simulink model "B5_simulation_paparazzi"  (R2021b)
settings: Solver=VariableStepAuto  StartTime=0.0  StopTime=5.5  FixedStep=0.002  RelTol=1e-3
values from neighbouring files (symbols this model uses):
  coef_sim_1 = tf_des_d.Denominator{1}(2)    [A11_setup_script_pprz.m]    (also in A1_setup_script.m; A6_slow_actuator.m)
  coef_sim_2 = tf_des_d.Numerator{1}(2)    [A11_setup_script_pprz.m]    (also in A1_setup_script.m; A6_slow_actuator.m)
  coeff = 1    [A11_setup_script_pprz.m]    (also in A12_sim_multi_run.m = coeff_list(i))
  doublet_mag = - 0.15    (= -0.15)    [A11_setup_script_pprz.m]    (also in A1_setup_script.m)
  doublet_time = 6    [A11_setup_script_pprz.m]    (also in A1_setup_script.m)
  f_8 = 1    [A11_setup_script_pprz.m]    (also in A1_setup_script.m)
  FILT_CUTOFF = 2*pi*5    (= 31.4159265359)    [A11_setup_script_pprz.m]    (also in A1_setup_script.m)
  FILTER = 1    [A11_setup_script_pprz.m]    (also in A1_setup_script.m)
  G1 = inv(I)*G1_r    [A10_simple_plant.m]    (also in A11_setup_script_pprz.m = G1/scale; A1_setup_script.m = [G1;G1_T])
  G2 = G2/scale    [A11_setup_script_pprz.m]    (also in A1_setup_script.m = (1/sampling_time)*inv(I)*(G2_r))
  h_plate = 0.3    [A11_setup_script_pprz.m]    (also in A1_setup_script.m = 0.16)
  I = eye(3,3)    [A10_simple_plant.m]    (also in A11_setup_script_pprz.m; A1_setup_script.m; A2_B_matrix_generation_symbolic.m = [Ixx 0 0; A3_B_matrix_generation_symbolic_cascaded.m = [Ixx 0 0)
  Iyy = 0.0008    [A11_setup_script_pprz.m]    (also in A1_setup_script.m = 0.0015)
  K = 7    [A11_setup_script_pprz.m]    (also in A1_setup_script.m = 10)
  K_act = 50    [A10_simple_plant.m]    (also in A11_setup_script_pprz.m = 20; A1_setup_script.m = 20)
  K_d = 15    [A11_setup_script_pprz.m]    (also in A1_setup_script.m = 25)
  K_dd = K_act    (= 20)    [A11_setup_script_pprz.m]    (also in A1_setup_script.m)
  K_ec = 50    [A11_setup_script_pprz.m]    (also in A1_setup_script.m = 251)
  K_ec_d = 13    [A11_setup_script_pprz.m]    (also in A1_setup_script.m = 25)
  K_ec_d_u = 1.5    [A11_setup_script_pprz.m]    (also in A1_setup_script.m = 5)
  K_ec_d_v = 1.5    [A11_setup_script_pprz.m]    (also in A1_setup_script.m = 5)
  K_ec_dd = 9    [A11_setup_script_pprz.m]    (also in A1_setup_script.m = 45)
  K_ec_i = 0    [A11_setup_script_pprz.m]    (also in A1_setup_script.m = 380)
  K_ec_u = 1.5    [A11_setup_script_pprz.m]    (also in A1_setup_script.m = 5)
  K_ec_v = 1.5    [A11_setup_script_pprz.m]    (also in A1_setup_script.m = 5)
  K_t = 0.0005    [A10_simple_plant.m]    (also in A11_setup_script_pprz.m = 6.557e-08; A1_setup_script.m = 6.557e-08)
  K_u = 1.0    (= 1)    [A11_setup_script_pprz.m]    (also in A1_setup_script.m = 1.5)
  K_u_d = 2.5    [A11_setup_script_pprz.m]    (also in A1_setup_script.m = 7)
  K_v = 1.0    (= 1)    [A11_setup_script_pprz.m]    (also in A1_setup_script.m = 1.5)
  K_v_d = 2.5    [A11_setup_script_pprz.m]    (also in A1_setup_script.m = 7)
  K_w = 1.0    (= 1)    [A11_setup_script_pprz.m]    (also in A1_setup_script.m = 4.5)
  K_w_d = 2.5    [A11_setup_script_pprz.m]    (also in A1_setup_script.m = 7)
  l_plate = 0.1    [A11_setup_script_pprz.m]    (also in A1_setup_script.m = 0.11)
  m = 0.4    [A10_simple_plant.m]    (also in A11_setup_script_pprz.m; A1_setup_script.m)
  NOISE = 0    [A11_setup_script_pprz.m]    (also in A1_setup_script.m)
  NOISE_ACC = 0.00005    (= 5e-05)    [A11_setup_script_pprz.m]    (also in A1_setup_script.m)
  NOISE_GYRO = 0.00005    (= 5e-05)    [A11_setup_script_pprz.m]    (also in A1_setup_script.m)
  NOISE_RPM = 200    [A11_setup_script_pprz.m]    (also in A1_setup_script.m)
  omega_des = 20.00    (= 20)    [A11_setup_script_pprz.m]    (also in A1_setup_script.m; A6_slow_actuator.m = 49)
  sampling_time = 1/frequency    (= 0.002)    [A11_setup_script_pprz.m]    (also in A12_sim_multi_run.m; A1_setup_script.m; A6_slow_actuator.m)
  scale_8 = 1.6    [A11_setup_script_pprz.m]    (also in A1_setup_script.m)
  start_8 = 2    [A11_setup_script_pprz.m]    (also in A1_setup_script.m)
  start_time = 2    [A11_setup_script_pprz.m]    (also in A1_setup_script.m = 1)
  t_8 = 10    [A11_setup_script_pprz.m]    (also in A1_setup_script.m)
  w_plate = 0.3    [A11_setup_script_pprz.m]    (also in A1_setup_script.m = 0.36)
undefined symbols (not defined in the file or in its folder): DiscIntNeverNeededParam
libraries: simulink x11, cstblocks x9, dspinverses x8, dspmathops x4, dspstat3 x4, aerolibutil x3, sharedutil x2, aerolibanim x1
(part 2 of 5)

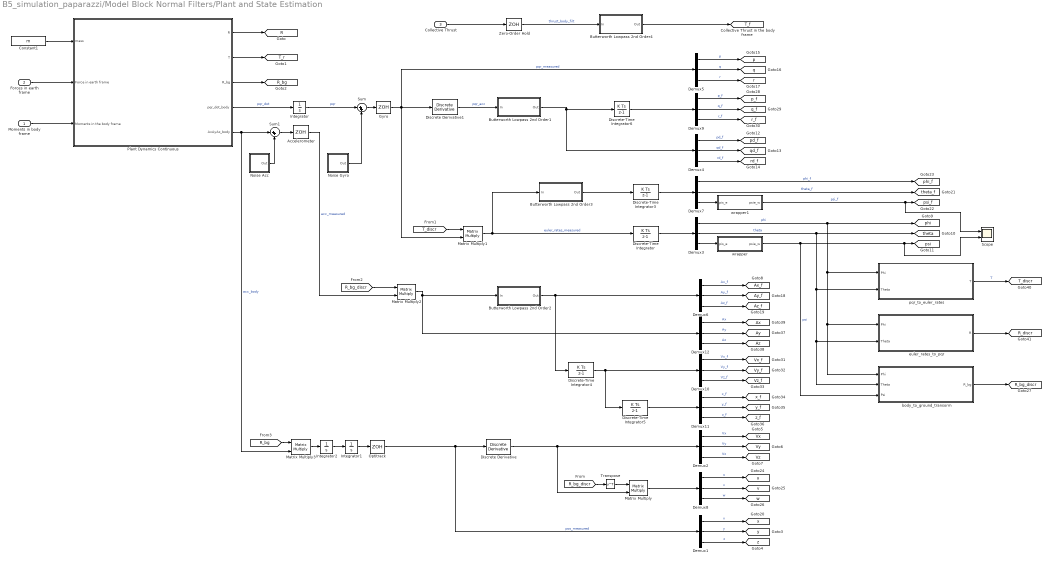
== system B5_simulation_paparazzi/Model Block Normal Filters/Plant and State Estimation ==
  Moments in body frame : Inport
  Forces in earth frame : Inport  Port=2
  Collective Thrust : Inport  Port=3
  Accelerometer : ZeroOrderHold  SampleTime=sampling_time
  Butterworth Lowpass 2nd Order1 : Subsystem
  Butterworth Lowpass 2nd Order2 : Subsystem
  Butterworth Lowpass 2nd Order3 : Subsystem
  Butterworth Lowpass 2nd Order4 : Subsystem
  Constant1 : Constant  Value=m  SampleTime=sampling_time
  Demux{1..12} (12 alike) : Demux  Outputs=3
  Discrete Derivative : simulink/Discrete/Discrete Derivative  gainval=1.0  ICPrevScaledInput=0.0  OutMin=[]  OutMax=[]  OutDataType=fixdt(1, 16)  OutScaling=2^-10  DoSatur=off
  Discrete Derivative1 : simulink/Discrete/Discrete Derivative  gainval=1.0  ICPrevScaledInput=0.0  OutMin=[]  OutMax=[]  OutDataType=fixdt(1, 16)  OutScaling=2^-10  DoSatur=off
  Discrete-Time Integrator{,3..5} (4 alike) : DiscreteIntegrator  SampleTime=sampling_time  ICPrevOutput=DiscIntNeverNeededParam  ICPrevScaledInput=DiscIntNeverNeededParam
  Discrete-Time Integrator6 : DiscreteIntegrator  SampleTime=-1  ICPrevOutput=DiscIntNeverNeededParam  ICPrevScaledInput=DiscIntNeverNeededParam
  Gyro : ZeroOrderHold  SampleTime=sampling_time
  Integrator : Integrator
  Integrator1 : Integrator
  Integrator2 : Integrator
  Matrix Multiply{,1..3} (4 alike) : Product  Multiplication=Matrix(*)
  Noise Acc : Subsystem
  Noise Gyro : Subsystem
  Optitrack : ZeroOrderHold  SampleTime=sampling_time
  Plant Dynamics Continuous : Subsystem
  Scope : Scope  NumInputPorts=2
  Sum : Sum  Inputs=|++
  Sum1 : Sum  Inputs=|++
  Transpose : Math  Operator=transpose  SaturateOnIntegerOverflow=on
  Zero-Order Hold : ZeroOrderHold  SampleTime=sampling_time
  body_to_ground_transorm : MATLAB Function  Description=|  TreatAsAtomicUnit=on
      | This function computes the rotational matrix to pass from the body frame to the world frame. 
      | Takes as inpout the euler angles.
  euler_rates_to_pqr : MATLAB Function  TreatAsAtomicUnit=on
  pqr_to_euler_rates : MATLAB Function  TreatAsAtomicUnit=on
  wrapper : MATLAB Function  TreatAsAtomicUnit=on
  wrapper1 : MATLAB Function  TreatAsAtomicUnit=on
  tag scope: Ax=global, Ax_f=global, Ay=global, Ay_f=global, Az=global, Az_f=global, R=global, R_bg=global, R_bg_discr=global, R_discr=global, T_discr=global, T_f=global, T_r=global, Vx=global, Vx_f=global, Vy=global, Vy_f=global, Vz=global, Vz_f=global, p=global, p_f=global, pd_f=global, phi=global, phi_f=global, psi=global, psi_f=global, q=global, q_f=global, qd_f=global, r=global, r_f=global, rd_f=global, theta=global, theta_f=global, u=global, v=global, w=global, x=global, x_f=global, y=global, y_f=global, z=global, z_f=global
  wires:
  Demux3/2 -> euler_rates_to_pqr/2(Theta), body_to_ground_transorm/2(Theta), pqr_to_euler_rates/2(Theta), [theta]  "theta"
  Demux4/1 -> [pd_f]  "pd_f"
  Demux3/1 -> body_to_ground_transorm/1(Phi), euler_rates_to_pqr/1(Phi), pqr_to_euler_rates/1(Phi), [phi]  "phi"
  Demux4/2 -> [qd_f]  "qd_f"
  Demux3/3 -> wrapper/1(pis_e)
  Discrete-Time Integrator/1 -> Demux3/1
  Demux5/2 -> [q]  "q"
  Demux5/1 -> [p]  "p"
  Plant Dynamics Continuous/4(pqr_dot_body) -> Integrator/1  "pqr_dot"
  Demux5/3 -> [r]  "r"
  Integrator/1 -> Sum/1  "pqr"
  Butterworth Lowpass 2nd Order1/1(Out) -> Demux4/1, Discrete-Time Integrator6/1
  Demux4/3 -> [rd_f]  "rd_f"
  Moments in body frame/1 -> Plant Dynamics Continuous/3(Moments in the body frame)
  Constant1/1 -> Plant Dynamics Continuous/1(mass)
  Forces in earth frame/1 -> Plant Dynamics Continuous/2(Force in earth frame)
  Plant Dynamics Continuous/1(R) -> [R]
  Plant Dynamics Continuous/2(T) -> [T_r]
  Plant Dynamics Continuous/3(R_bg) -> [R_bg]
  Demux2/2 -> [Vy]  "Vy"
  Demux6/2 -> [Ay_f]  "Ay_f"
  Discrete Derivative/1 -> Demux2/1, Matrix Multiply/2
  Demux6/1 -> [Ax_f]  "Ax_f"
  Accelerometer/1 -> Matrix Multiply2/2  "acc_measured"
  Demux2/1 -> [Vx]  "Vx"
  Demux1/2 -> [y]  "y"
  Demux1/1 -> [x]  "x"
  Demux1/3 -> [z]  "z"
  Demux6/3 -> [Az_f]  "Az_f"
  Demux2/3 -> [Vz]  "Vz"
  Plant Dynamics Continuous/5(AxAyAz_body) -> Matrix Multiply3/2, Sum1/1  "acc_body"
  Demux7/3 -> wrapper1/1(pis_e)
  Demux7/1 -> [phi_f]  "phi_f"
  Demux7/2 -> [theta_f]  "theta_f"
  Discrete-Time Integrator3/1 -> Demux7/1
  [R_bg_discr] -> Transpose/1
  Transpose/1 -> Matrix Multiply/1
  Demux8/2 -> [v]  "v"
  Demux8/1 -> [u]  "u"
  Demux8/3 -> [w]  "w"
  Matrix Multiply/1 -> Demux8/1
  Zero-Order Hold/1 -> Butterworth Lowpass 2nd Order4/1(In)  "thrust_body_filt"
  Collective Thrust/1 -> Zero-Order Hold/1
  Demux9/3 -> [r_f]  "r_f"
  Demux9/1 -> [p_f]  "p_f"
  Demux9/2 -> [q_f]  "q_f"
  Demux10/1 -> [Vx_f]  "Vx_f"
  Demux10/2 -> [Vy_f]  "Vy_f"
  Demux10/3 -> [Vz_f]  "Vz_f"
  Demux11/2 -> [y_f]  "y_f"
  Discrete-Time Integrator5/1 -> Demux11/1
  Demux11/1 -> [x_f]  "x_f"
  Demux11/3 -> [z_f]  "z_f"
  Discrete-Time Integrator4/1 -> Demux10/1, Discrete-Time Integrator5/1
  Demux12/2 -> [Ay]  "Ay"
  Demux12/1 -> [Ax]  "Ax"
  Demux12/3 -> [Az]  "Az"
  [T_discr] -> Matrix Multiply1/1
  Matrix Multiply1/1 -> Butterworth Lowpass 2nd Order3/1(In), Discrete-Time Integrator/1  "euler_rates_measured"
  euler_rates_to_pqr/1(R) -> [R_discr]
  pqr_to_euler_rates/1(T) -> [T_discr]  "T"
  body_to_ground_transorm/1(R_bg) -> [R_bg_discr]
  wrapper/1(psie_w) -> body_to_ground_transorm/3(Psi), Scope/2, [psi]  "psi"
  wrapper1/1(psie_w) -> Scope/1, [psi_f]  "psi_f"
  Sum/1 -> Gyro/1
  Sum1/1 -> Accelerometer/1
  Butterworth Lowpass 2nd Order2/1(Out) -> Discrete-Time Integrator4/1, Demux6/1
  [R_bg_discr] -> Matrix Multiply2/1
  Matrix Multiply2/1 -> Butterworth Lowpass 2nd Order2/1(In), Demux12/1
  Discrete Derivative1/1 -> Butterworth Lowpass 2nd Order1/1(In)  "pqr_acc"
  Discrete-Time Integrator6/1 -> Demux9/1
  Gyro/1 -> Demux5/1, Discrete Derivative1/1, Matrix Multiply1/2  "pqr_measured"
  Integrator1/1 -> Optitrack/1
  Integrator2/1 -> Integrator1/1
  Optitrack/1 -> Demux1/1, Discrete Derivative/1  "pos_measured"
  Matrix Multiply3/1 -> Integrator2/1
  [R_bg] -> Matrix Multiply3/1
  Noise Acc/1(Out) -> Sum1/2
  Noise Gyro/1(Out) -> Sum/2
  Butterworth Lowpass 2nd Order3/1(Out) -> Discrete-Time Integrator3/1
  Butterworth Lowpass 2nd Order4/1(Out) -> [T_f]

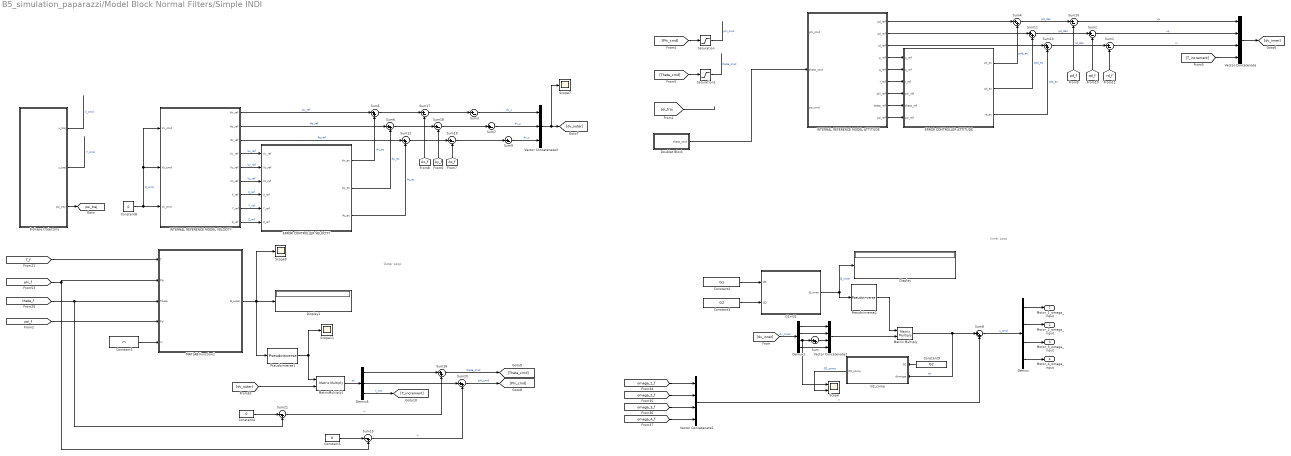
== system B5_simulation_paparazzi/Model Block Normal Filters/Simple INDI ==
  note: Inner Loop
  note: Outer Loop
  8-shape trajectory : Subsystem
  Constant1 : Constant  Value=m  SampleTime=sampling_time
  Constant2 : Constant  Value=G1  SampleTime=sampling_time
  Constant3 : Constant  Value=G2  SampleTime=sampling_time
  Constant4 : Constant  Value=0
  Constant5 : Constant  Value=0
  Constant8 : Constant  Value=0  SampleTime=sampling_time
  Constant9 : Constant  Value=G2  SampleTime=sampling_time
  Demux : Demux
  Demux1 : Demux
  Demux5 : Demux  Outputs=3
  Display : Display
  Display1 : Display
  Doublet Block : Subsystem
  ERROR CONTROLLER ATTITUDE : Subsystem
  ERROR CONTROLLER VELOCITY : Subsystem
  G1+G2 : MATLAB Function  TreatAsAtomicUnit=on
  G2_comp : MATLAB Function  TreatAsAtomicUnit=on
  INTERNAL REFERENCE MODEL ATTITUDE : Subsystem
  INTERNAL REFERENCE MODEL VELOCITY : Subsystem
  MATLAB Function1 : MATLAB Function  TreatAsAtomicUnit=on
  Matrix Multiply : Product  Multiplication=Matrix(*)
  MatrixMultiply1 : Product  Multiplication=Matrix(*)
  Pseudoinverse1 : dspinverses/Pseudoinverse  wanterr=off  SimulateUsing=Interpreted execution
      settings: SourceProductBaseCode=DS
  Pseudoinverse2 : dspinverses/Pseudoinverse  wanterr=off  SimulateUsing=Interpreted execution
      settings: SourceProductBaseCode=DS
  Saturation : Saturate
  Saturation1 : Saturate
  Scope : Scope  NumInputPorts=2
  Scope11 : Scope
  Scope7 : Scope
  Scope9 : Scope
  Sum{,4..6,8,11..13,16,20} (10 alike) : Sum  Inputs=|++
  Sum{1..3,7,9..10,17..19} (9 alike) : Sum  Inputs=|+-
  Sum15 : Sum  Inputs=|-+
  Sum21 : Sum  Inputs=|-+
  Vector Concatenate : Concatenate  NumInputs=4
  Vector Concatenate1 : Concatenate  NumInputs=4
  Vector Concatenate2 : Concatenate  NumInputs=4
  Vector Concatenate3 : Concatenate  NumInputs=3
  Motor_1_omega_input : Outport
  Motor_2_omega_input : Outport  Port=2
  Motor_3_omega_input : Outport  Port=3
  Motor_4_omega_input : Outport  Port=4
  tag scope: psi_traj=global
  wires:
  G1+G2/1(B_inner) -> Pseudoinverse2/1, Display/1  "B_inner"
  Vector Concatenate1/1 -> Sum8/2  "u"
  Vector Concatenate/1 -> [dv_inner]
  Matrix Multiply/1 -> G2_comp/2(domega), Sum8/1  "du"
  Demux/1 -> Motor_1_omega_input/1
  [omega_4_f] -> Vector Concatenate1/4
  [omega_2_f] -> Vector Concatenate1/2
  Demux/3 -> Motor_3_omega_input/1
  Sum8/1 -> Demux/1  "u_cmd"
  Pseudoinverse2/1 -> Matrix Multiply/1
  [omega_1_f] -> Vector Concatenate1/1
  Demux/2 -> Motor_2_omega_input/1
  Demux/4 -> Motor_4_omega_input/1
  [omega_3_f] -> Vector Concatenate1/3
  INTERNAL REFERENCE MODEL VELOCITY/5(Vy_ref) -> ERROR CONTROLLER VELOCITY/2(Vy_ref)  "Vy_ref"
  Constant4/1 -> Sum21/1
  Sum16/1 -> [Theta_cmd]  "theta_cmd"
  Sum9/1 -> Vector Concatenate3/3  "dv_z"
  INTERNAL REFERENCE MODEL VELOCITY/2(Ay_ref) -> Sum6/1  "Ay_ref"
  Sum21/1 -> Sum16/2  "u"
  INTERNAL REFERENCE MODEL VELOCITY/6(Vz_ref) -> ERROR CONTROLLER VELOCITY/3(Vz_ref)  "Vz_ref"
  INTERNAL REFERENCE MODEL VELOCITY/4(Vx_ref) -> ERROR CONTROLLER VELOCITY/1(Vx_ref)  "Vx_ref"
  ERROR CONTROLLER VELOCITY/2(Ay_ec) -> Sum6/2  "Ay_ec"
  8-shape trajectory/1(x_traj) -> ?  "X_cmd"
  Sum7/1 -> Vector Concatenate3/2  "dv_y"
  ERROR CONTROLLER VELOCITY/1(Ax_ec) -> Sum5/2  "Ax_ec"
  Sum3/1 -> Vector Concatenate3/1  "dv_x"
  ERROR CONTROLLER VELOCITY/3(Az_ec) -> Sum12/2  "Az_ec"
  Sum12/1 -> Sum19/1
  Constant8/1 -> INTERNAL REFERENCE MODEL VELOCITY/1(Vx_cmd), INTERNAL REFERENCE MODEL VELOCITY/2(Vy_cmd), INTERNAL REFERENCE MODEL VELOCITY/3(Vz_cmd)  "Z_cmd"
  Pseudoinverse1/1 -> Scope11/1, MatrixMultiply1/1
  Sum15/1 -> Sum20/2  "u"
  Vector Concatenate3/1 -> Scope7/1, [dv_outer]
  INTERNAL REFERENCE MODEL VELOCITY/1(Ax_ref) -> Sum5/1  "Ax_ref"
  INTERNAL REFERENCE MODEL VELOCITY/3(Az_ref) -> Sum12/1  "Az_ref"
  Sum20/1 -> [Phi_cmd]  "phi_cmd"
  [T_f] -> MATLAB Function1/1(T)
  Sum6/1 -> Sum18/1
  Constant5/1 -> Sum15/1
  [dv_outer] -> MatrixMultiply1/2
  MATLAB Function1/1(B_outer) -> Scope9/1, Display1/1, Pseudoinverse1/1
  Demux5/3 -> [T_increment]  "t_incr"
  MatrixMultiply1/1 -> Demux5/1  "du"
  8-shape trajectory/2(y_traj) -> ?  "Y_cmd"
  [Ax_f] -> Sum17/2
  [Ay_f] -> Sum18/2
  [Az_f] -> Sum19/2
  [Phi_cmd] -> Saturation/1
  [theta_f] -> Sum21/2, MATLAB Function1/3(Theta)
  [phi_f] -> Sum15/2, MATLAB Function1/2(Phi)
  INTERNAL REFERENCE MODEL ATTITUDE/4(p_ref) -> ERROR CONTROLLER ATTITUDE/1(p_ref)
  ERROR CONTROLLER ATTITUDE/3(rd_ec) -> Sum13/2  "rdd_ec"
  ERROR CONTROLLER ATTITUDE/2(qd_ec) -> Sum11/2  "qdd_ec"
  INTERNAL REFERENCE MODEL ATTITUDE/8(theta_ref) -> ERROR CONTROLLER ATTITUDE/5(theta_ref)
  INTERNAL REFERENCE MODEL ATTITUDE/5(q_ref) -> ERROR CONTROLLER ATTITUDE/2(q_ref)
  ERROR CONTROLLER ATTITUDE/1(pd_ec) -> Sum4/2  "pdd_ec"
  INTERNAL REFERENCE MODEL ATTITUDE/7(phi_ref) -> ERROR CONTROLLER ATTITUDE/4(phi_ref)
  INTERNAL REFERENCE MODEL ATTITUDE/9(psi_ref) -> ERROR CONTROLLER ATTITUDE/6(psi_ref)
  INTERNAL REFERENCE MODEL ATTITUDE/6(r_ref) -> ERROR CONTROLLER ATTITUDE/3(r_ref)
  [T_increment] -> Vector Concatenate/4
  Constant3/1 -> G1+G2/2(G2)
  Constant2/1 -> G1+G2/1(G1)
  Constant9/1 -> G2_comp/1(G2)
  [dv_inner] -> Demux1/1  "dv_inner"
  Sum/1 -> Vector Concatenate2/3
  Demux1/3 -> Scope/1, Sum/1
  Demux1/2 -> Vector Concatenate2/2
  Demux1/1 -> Vector Concatenate2/1
  Demux1/4 -> Vector Concatenate2/4
  Vector Concatenate2/1 -> Matrix Multiply/2
  G2_comp/1(G2_comp) -> Scope/2  "G2_comp"
  Sum5/1 -> Sum17/1
  Saturation1/1 -> ?  "theta_cmd"
  8-shape trajectory/3(psi_traj) -> [psi_traj]
  [Theta_cmd] -> Saturation1/1
  Saturation/1 -> ?  "phi_cmd"
  Sum17/1 -> Sum3/1
  Sum18/1 -> Sum7/1
  Sum19/1 -> Sum9/1
  Constant1/1 -> MATLAB Function1/5(m)
  Demux5/2 -> Sum20/1
  Demux5/1 -> Sum16/1
  [psi_f] -> MATLAB Function1/4(Psi)
  [psi_traj] -> ?
  INTERNAL REFERENCE MODEL VELOCITY/7(X_ref) -> ERROR CONTROLLER VELOCITY/4(X_ref)  "X_ref"
  INTERNAL REFERENCE MODEL VELOCITY/8(Y_ref) -> ERROR CONTROLLER VELOCITY/5(Y_ref)  "Y_ref"
  INTERNAL REFERENCE MODEL VELOCITY/9(Z_ref) -> ERROR CONTROLLER VELOCITY/6(Z_ref)  "Z_ref"
  Doublet Block/1(theta_cmd) -> INTERNAL REFERENCE MODEL ATTITUDE/2(theta_cmd)
  INTERNAL REFERENCE MODEL ATTITUDE/3(rd_ref) -> Sum13/1
  INTERNAL REFERENCE MODEL ATTITUDE/2(qd_ref) -> Sum11/1
  INTERNAL REFERENCE MODEL ATTITUDE/1(pd_ref) -> Sum4/1
  Sum11/1 -> Sum2/1  "qd_des"
  Sum4/1 -> Sum10/1  "pd_des"
  Sum10/1 -> Vector Concatenate/1  "vp"
  Sum2/1 -> Vector Concatenate/2  "vq"
  Sum1/1 -> Vector Concatenate/3  "vr"
  Sum13/1 -> Sum1/1  "rd_des"
  [pd_f] -> Sum10/2
  [qd_f] -> Sum2/2
  [rd_f] -> Sum1/2

== system B5_simulation_paparazzi/Model Block Complementary Filters/Continuous Actuator Dynamics/Noise RPM ==
  Constant : Constant  Value=NOISE  SampleTime=sampling_time
  Merge : Merge
  Switch Case : SwitchCase
  Switch Case Action Subsystem : Subsystem  TreatAsAtomicUnit=on
  Switch Case Action Subsystem1 : Subsystem  TreatAsAtomicUnit=on
  Out : Outport
  wires:
  Switch Case/2 -> Switch Case Action Subsystem1/Action
  Merge/1 -> Out/1
  Switch Case/1 -> Switch Case Action Subsystem/Action
  Constant/1 -> Switch Case/1
  Switch Case Action Subsystem1/1(Out1) -> Merge/2
  Switch Case Action Subsystem/1(Out1) -> Merge/1

== system B5_simulation_paparazzi/Model Block Complementary Filters/Extended INDI/8-shape trajectory ==
  Abs : Abs
  Abs1 : Abs
  Clock : Clock
      settings: Decimation=100
  Constant : Constant  Value=f_8
  Constant1 : Constant  Value=scale_8
  Constant2 : Constant  Value=t_8
  Constant3 : Constant  Value=sampling_time
  Constant4 : Constant  Value=0
  Constant5 : Constant  Value=start_8
  Constant6 : Constant  Value=t_8
  Constant7 : Constant  Value=start_8
  Integrator : Integrator
  MATLAB Function : MATLAB Function  TreatAsAtomicUnit=on
  Scope : Scope
  Scope1 : Scope
  Sum : Sum  Inputs=|+-
  Sum3 : Sum  Inputs=|+-
  Sum7 : Sum  Inputs=|+-
  Sum9 : Sum  Inputs=|++
  Switch : Switch  Criteria=u2 > Threshold  Threshold=t_8
  Switch1 : Switch  Criteria=u2 > Threshold  Threshold=start_8
  Zero-Order Hold : ZeroOrderHold  SampleTime=sampling_time
  x_traj : Outport
  y_traj : Outport  Port=2
  psi_traj : Outport  Port=3
  wires:
  Constant2/1 -> Switch/1
  Switch/1 -> Scope/1, MATLAB Function/1(t)  "t"
  Constant/1 -> MATLAB Function/2(f)
  MATLAB Function/2(y) -> y_traj/1, Sum7/2  "y_traj"
  Zero-Order Hold/1 -> Switch/2, Switch/3
  Constant1/1 -> MATLAB Function/3(scale)
  Constant3/1 -> MATLAB Function/4(sampling_time)
  MATLAB Function/1(x) -> x_traj/1, Sum3/2  "x_traj"
  MATLAB Function/3(psi) -> psi_traj/1  "psi_traj"
  Clock/1 -> Sum/1, Switch1/2
  Constant4/1 -> Switch1/3
  Switch1/1 -> Zero-Order Hold/1
  Constant5/1 -> Sum/2
  Sum/1 -> Switch1/1
  Constant6/1 -> MATLAB Function/5(total_time)
  Sum7/1 -> Abs1/1
  Abs/1 -> Sum9/1
  Abs1/1 -> Sum9/2
  [y] -> Sum7/1
  Sum9/1 -> Integrator/1
  Integrator/1 -> Scope1/1  "pos_err"
  [x] -> Sum3/1
  Sum3/1 -> Abs/1
  Constant7/1 -> MATLAB Function/6(start_time)

== system B5_simulation_paparazzi/Model Block Complementary Filters/Extended INDI/Doublet Block ==
  Scope : Scope
  Step : Step  Time=start_time  After=doublet_mag  SampleTime=sampling_time
  theta_cmd : Outport
  wires:
  Step/1 -> theta_cmd/1, Scope/1

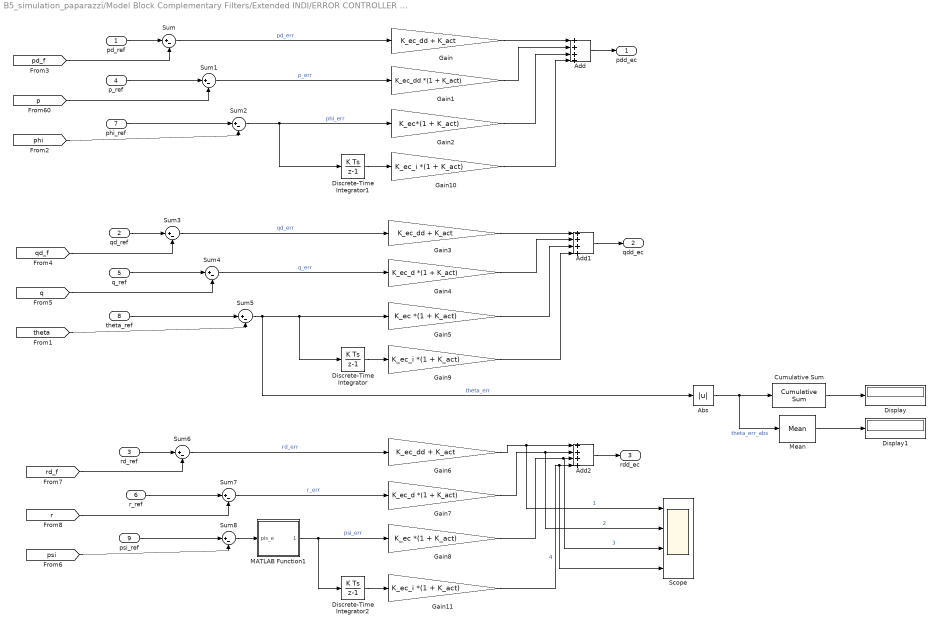
== system B5_simulation_paparazzi/Model Block Complementary Filters/Extended INDI/ERROR CONTROLLER ATTITUDE ==
  pd_ref : Inport
  qd_ref : Inport  Port=2
  rd_ref : Inport  Port=3
  p_ref : Inport  Port=4
  q_ref : Inport  Port=5
  r_ref : Inport  Port=6
  phi_ref : Inport  Port=7
  theta_ref : Inport  Port=8
  psi_ref : Inport  Port=9
  Abs : Abs
  Add : Sum  Inputs=++++
  Add1 : Sum  Inputs=++++
  Add2 : Sum  Inputs=++++
  Cumulative Sum : dspmathops/Cumulative Sum  dim=Channels (running sum)  InputProcessing=Columns as channels (frame based)  reset_popup=None  roundingMode=Floor  overflowMode=off  outputDataTypeStr=Inherit: Same as accumulator  outputMin=[]  outputMax=[]  outputLastDataTypeStr=Inherit: Same as accumulator
  Discrete-Time Integrator : DiscreteIntegrator  SampleTime=-1  ICPrevOutput=DiscIntNeverNeededParam  ICPrevScaledInput=DiscIntNeverNeededParam
  Discrete-Time Integrator1 : DiscreteIntegrator  SampleTime=-1  ICPrevOutput=DiscIntNeverNeededParam  ICPrevScaledInput=DiscIntNeverNeededParam
  Discrete-Time Integrator2 : DiscreteIntegrator  SampleTime=-1  ICPrevOutput=DiscIntNeverNeededParam  ICPrevScaledInput=DiscIntNeverNeededParam
  Display : Display
  Display1 : Display
  Gain : Gain  Gain=K_ec_dd + K_act
  Gain1 : Gain  Gain=K_ec_dd *(1 + K_act)
  Gain10 : Gain  Gain=K_ec_i *(1 + K_act)
  Gain11 : Gain  Gain=K_ec_i *(1 + K_act)
  Gain2 : Gain  Gain=K_ec*(1 + K_act)
  Gain3 : Gain  Gain=K_ec_dd + K_act
  Gain4 : Gain  Gain=K_ec_d *(1 + K_act)
  Gain5 : Gain  Gain=K_ec *(1 + K_act)
  Gain6 : Gain  Gain=K_ec_dd + K_act
  Gain7 : Gain  Gain=K_ec_d *(1 + K_act)
  Gain8 : Gain  Gain=K_ec *(1 + K_act)
  Gain9 : Gain  Gain=K_ec_i *(1 + K_act)
  MATLAB Function1 : MATLAB Function  TreatAsAtomicUnit=on
  Mean : dspstat3/Mean  run=off  InputProcessing=Columns as channels (frame based)  reset_popup=None  directionMode=Each column  dimension=1  roiEnable=off  roiType=Rectangles  roiPortion=Entire ROI  roiOutput=Individual statistics for each ROI  roiFlag=off  roundingMode=Floor  overflowMode=off  outputDataTypeStr=Inherit: Same as accumulator  outputMin=[]  outputMax=[]  outputLastDataTypeStr=Inherit: Same as accumulator
  Scope : Scope  NumInputPorts=4
  Sum{,1..8} (9 alike) : Sum  Inputs=|+-
  pdd_ec : Outport
  qdd_ec : Outport  Port=2
  rdd_ec : Outport  Port=3
  wires:
  pd_ref/1 -> Sum/1
  p_ref/1 -> Sum1/1
  Add/1 -> pdd_ec/1
  [p] -> Sum1/2
  [phi] -> Sum2/2
  phi_ref/1 -> Sum2/1
  [pd_f] -> Sum/2
  Sum/1 -> Gain/1  "pd_err"
  Gain/1 -> Add/1
  Sum1/1 -> Gain1/1  "p_err"
  Sum2/1 -> Discrete-Time Integrator1/1, Gain2/1  "phi_err"
  Gain1/1 -> Add/2
  Gain2/1 -> Add/3
  Sum4/1 -> Gain4/1  "q_err"
  [qd_f] -> Sum3/2
  Gain4/1 -> Add1/2
  Gain5/1 -> Add1/3
  theta_ref/1 -> Sum5/1
  [theta] -> Sum5/2
  [q] -> Sum4/2
  Gain3/1 -> Add1/1
  q_ref/1 -> Sum4/1
  Add1/1 -> qdd_ec/1
  qd_ref/1 -> Sum3/1
  Sum7/1 -> Gain7/1  "r_err"
  Sum8/1 -> MATLAB Function1/1(pis_e)
  Sum6/1 -> Gain6/1  "rd_err"
  [rd_f] -> Sum6/2
  Gain7/1 -> Scope/2, Add2/2  "2"
  Gain8/1 -> Scope/3, Add2/3  "3"
  psi_ref/1 -> Sum8/1
  [psi] -> Sum8/2
  [r] -> Sum7/2
  Gain6/1 -> Add2/1, Scope/1  "1"
  r_ref/1 -> Sum7/1
  Add2/1 -> rdd_ec/1
  rd_ref/1 -> Sum6/1
  Sum3/1 -> Gain3/1  "qd_err"
  Sum5/1 -> Abs/1, Discrete-Time Integrator/1, Gain5/1  "theta_err"
  MATLAB Function1/1(psie_w) -> Discrete-Time Integrator2/1, Gain8/1  "psi_err"
  Abs/1 -> Mean/1, Cumulative Sum/1  "theta_err_abs"
  Cumulative Sum/1 -> Display/1
  Mean/1 -> Display1/1
  Discrete-Time Integrator/1 -> Gain9/1
  Gain9/1 -> Add1/4
  Discrete-Time Integrator1/1 -> Gain10/1
  Gain10/1 -> Add/4
  Discrete-Time Integrator2/1 -> Gain11/1
  Gain11/1 -> Scope/4, Add2/4  "4"

== system B5_simulation_paparazzi/Model Block Complementary Filters/Extended INDI/ERROR CONTROLLER VELOCITY ==
  Vx_ref : Inport
  Vy_ref : Inport  Port=2
  Vz_ref : Inport  Port=3
  X_ref : Inport  Port=4
  Y_ref : Inport  Port=5
  Z_ref : Inport  Port=6
  Gain : Gain  Gain=K_ec_u
  Gain1 : Gain  Gain=K_ec_d_u
  Gain2 : Gain  Gain=K_ec_v
  Gain3 : Gain  Gain=K_ec_d_v
  Gain4 : Gain  Gain=K_ec_v
  Gain5 : Gain  Gain=K_ec_d_v
  Sum{,3,5..8} (6 alike) : Sum  Inputs=|+-
  Sum1 : Sum  Inputs=|++
  Sum2 : Sum  Inputs=|++
  Sum4 : Sum  Inputs=|++
  Ax_ec : Outport
  Ay_ec : Outport  Port=2
  Az_ec : Outport  Port=3
  wires:
  [Vz] -> Sum6/2
  Sum1/1 -> Ax_ec/1
  Sum2/1 -> Ay_ec/1
  Vy_ref/1 -> Sum3/1
  Vx_ref/1 -> Sum/1
  [Vy] -> Sum3/2
  Vz_ref/1 -> Sum6/1
  Sum/1 -> Gain1/1  "Vx_error"
  Sum4/1 -> Az_ec/1
  [Vx] -> Sum/2
  [x] -> Sum5/2
  X_ref/1 -> Sum5/1
  Sum5/1 -> Gain/1
  Gain1/1 -> Sum1/1
  Gain/1 -> Sum1/2
  Gain3/1 -> Sum2/1
  Sum3/1 -> Gain3/1  "Vy_error"
  Gain5/1 -> Sum4/1
  Sum6/1 -> Gain5/1  "Vz_error"
  Y_ref/1 -> Sum7/1
  [y] -> Sum7/2
  Sum7/1 -> Gain2/1
  Z_ref/1 -> Sum8/1
  [z] -> Sum8/2
  Sum8/1 -> Gain4/1
  Gain4/1 -> Sum4/2
  Gain2/1 -> Sum2/2

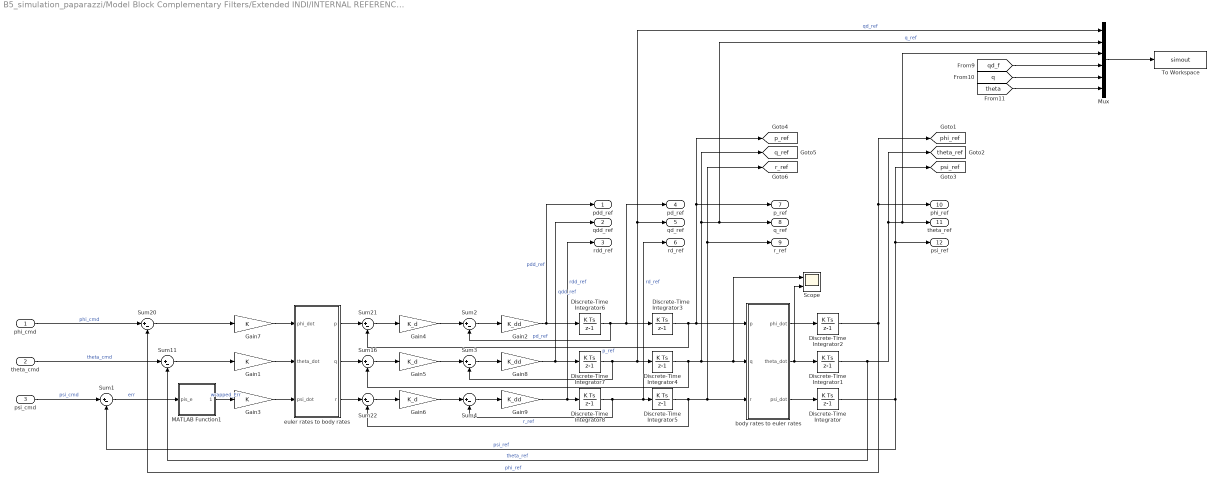
== system B5_simulation_paparazzi/Model Block Complementary Filters/Extended INDI/INTERNAL REFERENCE MODEL ATTITUDE ==
  phi_cmd : Inport
  theta_cmd : Inport  Port=2
  psi_cmd : Inport  Port=3
  Discrete-Time Integrator{,1..8} (9 alike) : DiscreteIntegrator  SampleTime=sampling_time  ICPrevOutput=DiscIntNeverNeededParam  ICPrevScaledInput=DiscIntNeverNeededParam
  Gain1 : Gain  Gain=K
  Gain2 : Gain  Gain=K_dd
  Gain3 : Gain  Gain=K
  Gain4 : Gain  Gain=K_d
  Gain5 : Gain  Gain=K_d
  Gain6 : Gain  Gain=K_d
  Gain7 : Gain  Gain=K
  Gain8 : Gain  Gain=K_dd
  Gain9 : Gain  Gain=K_dd
  MATLAB Function1 : MATLAB Function  TreatAsAtomicUnit=on
  Mux : Mux  Inputs=6
  Scope : Scope  NumInputPorts=2
  Sum{1..4,11,16,20..22} (9 alike) : Sum  Inputs=|+-
  To Workspace : ToWorkspace  VariableName=simout  SaveFormat=Timeseries  SampleTime=-1
  body rates to euler rates : Subsystem
  euler rates to body rates : Subsystem
  pdd_ref : Outport
  qdd_ref : Outport  Port=2
  rdd_ref : Outport  Port=3
  pd_ref : Outport  Port=4
  qd_ref : Outport  Port=5
  rd_ref : Outport  Port=6
  p_ref : Outport  Port=7
  q_ref : Outport  Port=8
  r_ref : Outport  Port=9
  phi_ref : Outport  Port=10
  theta_ref : Outport  Port=11
  psi_ref : Outport  Port=12
  tag scope: p_ref=global, phi_ref=global, psi_ref=global, q_ref=global, r_ref=global, theta_ref=global
  wires:
  Discrete-Time Integrator1/1 -> [theta_ref], Mux/3, theta_ref/1, Sum11/2  "theta_ref"
  Discrete-Time Integrator8/1 -> Sum4/2, Discrete-Time Integrator5/1, rd_ref/1  "rd_ref"
  Discrete-Time Integrator3/1 -> [p_ref], p_ref/1, body rates to euler rates/1(p), Sum21/2  "p_ref"
  Discrete-Time Integrator5/1 -> [r_ref], r_ref/1, body rates to euler rates/3(r), Sum22/2  "r_ref"
  Discrete-Time Integrator4/1 -> Scope/1, body rates to euler rates/2(q), [q_ref], Mux/2, q_ref/1, Sum16/2  "q_ref"
  Discrete-Time Integrator7/1 -> Sum3/2, Discrete-Time Integrator4/1, Mux/1, qd_ref/1  "qd_ref"
  Sum21/1 -> Gain4/1
  Sum11/1 -> Gain1/1
  Sum22/1 -> Gain6/1
  Sum16/1 -> Gain5/1
  Discrete-Time Integrator2/1 -> [phi_ref], phi_ref/1, Sum20/2  "phi_ref"
  Sum20/1 -> Gain7/1
  Discrete-Time Integrator6/1 -> Sum2/2, Discrete-Time Integrator3/1, pd_ref/1  "pd_ref"
  phi_cmd/1 -> Sum20/1  "phi_cmd"
  theta_cmd/1 -> Sum11/1  "theta_cmd"
  psi_cmd/1 -> Sum1/1  "psi_cmd"
  Discrete-Time Integrator/1 -> [psi_ref], psi_ref/1, Sum1/2  "psi_ref"
  Sum1/1 -> MATLAB Function1/1(pis_e)  "err"
  Gain4/1 -> Sum2/1
  Gain5/1 -> Sum3/1
  Gain6/1 -> Sum4/1
  Sum2/1 -> Gain2/1
  Sum3/1 -> Gain8/1
  Sum4/1 -> Gain9/1
  Gain2/1 -> Discrete-Time Integrator6/1, pdd_ref/1  "pdd_ref"
  Gain8/1 -> Discrete-Time Integrator7/1, qdd_ref/1  "qdd_ref"
  Gain9/1 -> Discrete-Time Integrator8/1, rdd_ref/1  "rdd_ref"
  Gain7/1 -> euler rates to body rates/1(phi_dot)
  euler rates to body rates/1(p) -> Sum21/1
  Gain1/1 -> euler rates to body rates/2(theta_dot)
  euler rates to body rates/2(q) -> Sum16/1
  Gain3/1 -> euler rates to body rates/3(psi_dot)
  euler rates to body rates/3(r) -> Sum22/1
  body rates to euler rates/3(psi_dot) -> Discrete-Time Integrator/1
  body rates to euler rates/2(theta_dot) -> Scope/2, Discrete-Time Integrator1/1
  body rates to euler rates/1(phi_dot) -> Discrete-Time Integrator2/1
  MATLAB Function1/1(psie_w) -> Gain3/1  "wrapped_Err"
  Mux/1 -> To Workspace/1
  [qd_f] -> Mux/4
  [q] -> Mux/5
  [theta] -> Mux/6

== system B5_simulation_paparazzi/Model Block Complementary Filters/Extended INDI/INTERNAL REFERENCE MODEL VELOCITY ==
  Vx_cmd : Inport
  Vy_cmd : Inport  Port=2
  Vz_cmd : Inport  Port=3
  Discrete-Time Integrator{,1..5} (6 alike) : DiscreteIntegrator  SampleTime=-1  ICPrevOutput=DiscIntNeverNeededParam  ICPrevScaledInput=DiscIntNeverNeededParam
  Gain1 : Gain  Gain=K_w_d
  Gain2 : Gain  Gain=K_v_d
  Gain3 : Gain  Gain=K_w
  Gain4 : Gain  Gain=K_v
  Gain5 : Gain  Gain=K_u
  Gain9 : Gain  Gain=K_u_d
  Sum{1..4,11,20} (6 alike) : Sum  Inputs=|+-
  Ax_ref : Outport
  Ay_ref : Outport  Port=2
  Az_ref : Outport  Port=3
  Vx_ref : Outport  Port=4
  Vy_ref : Outport  Port=5
  Vz_ref : Outport  Port=6
  X_ref : Outport  Port=7
  Y_ref : Outport  Port=8
  Z_ref : Outport  Port=9
  tag scope: Ax_ref=global, Ay_ref=global, Az_ref=global, Vx_ref=global, Vy_ref=global, Vz_ref=global
  wires:
  Discrete-Time Integrator1/1 -> Sum3/2, Discrete-Time Integrator4/1, [Vy_ref], Vz_ref/1
  Gain1/1 -> Discrete-Time Integrator1/1, [Az_ref], Az_ref/1
  Gain9/1 -> Discrete-Time Integrator/1, [Ax_ref], Ax_ref/1
  Vy_cmd/1 -> Sum1/1
  Discrete-Time Integrator/1 -> Sum4/2, Discrete-Time Integrator3/1, [Vx_ref], Vx_ref/1
  Vx_cmd/1 -> Sum20/1
  Vz_cmd/1 -> Sum11/1
  Discrete-Time Integrator2/1 -> Sum2/2, Discrete-Time Integrator5/1, [Vz_ref], Vy_ref/1
  Gain2/1 -> Discrete-Time Integrator2/1, [Ay_ref], Ay_ref/1
  Sum20/1 -> Gain5/1
  Sum11/1 -> Gain3/1
  Sum1/1 -> Gain4/1
  Gain4/1 -> Sum2/1
  Gain3/1 -> Sum3/1
  Gain5/1 -> Sum4/1
  Sum3/1 -> Gain1/1
  Sum2/1 -> Gain2/1
  Sum4/1 -> Gain9/1
  Discrete-Time Integrator3/1 -> X_ref/1, Sum20/2
  Discrete-Time Integrator4/1 -> Sum11/2, Z_ref/1
  Discrete-Time Integrator5/1 -> Sum1/2, Y_ref/1

== system B5_simulation_paparazzi/Model Block Complementary Filters/Extended INDI/Subsystem ==
  Constant : Constant  Value=w_plate
  Constant1 : Constant  Value=Iyy
  Constant2 : Constant  Value=l_plate
  Constant3 : Constant  Value=h_plate
  MATLAB Function : MATLAB Function  TreatAsAtomicUnit=on
  Terminator : Terminator
  Terminator1 : Terminator
  body rates to euler rates : Subsystem
  qdd_comp : Outport
  wires:
  MATLAB Function/1(qdd_comp) -> qdd_comp/1  "qdd_comp"
  [theta] -> MATLAB Function/1(theta)
  [Vx] -> MATLAB Function/3(Vx)
  [Ax] -> MATLAB Function/6(Ax)
  Constant/1 -> MATLAB Function/10(w_plate)
  Constant1/1 -> MATLAB Function/13(Iyy)
  Constant2/1 -> MATLAB Function/12(l_plate)
  Constant3/1 -> MATLAB Function/11(h_plate)
  [p] -> body rates to euler rates/1(p)
  [q] -> body rates to euler rates/2(q)
  [r] -> body rates to euler rates/3(r)
  body rates to euler rates/2(theta_dot) -> MATLAB Function/2(dtheta)
  body rates to euler rates/1(phi_dot) -> Terminator/1
  [Vy] -> MATLAB Function/4(Vy)
  [Ay] -> MATLAB Function/7(Ay)
  body rates to euler rates/3(psi_dot) -> Terminator1/1
  [u] -> MATLAB Function/9(u)
  [Vz] -> MATLAB Function/5(Vz)
  [Az] -> MATLAB Function/8(Az)

== system B5_simulation_paparazzi/Model Block Complementary Filters/Force and Moment Calculation/Drag Plate Aerodynamics ==
  Constant : Constant  Value=0  SampleTime=sampling_time
  Constant1 : Constant  Value=w_plate
  Constant4 : Constant  Value=h_plate
  Constant6 : Constant  Value=l_plate
  Mux : Mux  Inputs=3
  Scope1 : Scope  NumInputPorts=3
  Scope2 : Scope  NumInputPorts=2
  Scope3 : Scope  NumInputPorts=3
  Scope4 : Scope
  Scope5 : Scope  NumInputPorts=3
  drag plate My1 : MATLAB Function  TreatAsAtomicUnit=on
  aero_moment : Outport
  wires:
  Constant4/1 -> drag plate My1/2(h_plate)
  Constant6/1 -> drag plate My1/3(l_plate)
  [theta_cont] -> drag plate My1/4("theta ")
  Constant1/1 -> drag plate My1/1(w_plate)
  [Vy_cont] -> drag plate My1/6("Vy ")
  [Vx_cont] -> drag plate My1/5("Vx ")
  drag plate My1/6(gamma) -> Scope1/1  "gamma"
  [Vz_cont] -> drag plate My1/7("Vz ")
  drag plate My1/7(theta) -> Scope1/2  "theta_deg"
  drag plate My1/8(alpha) -> Scope1/3  "alpha"
  drag plate My1/1(Cd) -> Scope2/1  "Cd"
  drag plate My1/2(Cl) -> Scope2/2  "Cl"
  drag plate My1/9(D_plate) -> Scope3/1  "D_plate"
  drag plate My1/10(L_plate) -> Scope3/2  "L_plate"
  [u_cont] -> drag plate My1/8(u)
  drag plate My1/12(My_dp) -> Mux/2, Scope4/1  "My_dp"
  drag plate My1/3(Vx) -> Scope5/1  "Vx"
  drag plate My1/4(Vy) -> Scope5/2  "Vy"
  drag plate My1/5(Vz) -> Scope5/3  "Vz"
  Constant/1 -> Mux/1, Mux/3
  Mux/1 -> aero_moment/1
  drag plate My1/11(R_plate) -> Scope3/3  "R_plate"

== system B5_simulation_paparazzi/Model Block Complementary Filters/Plant and State Estimation/Angular Velocity Model ==
  Constant1 : Constant  Value=sampling_time  SampleTime=sampling_time
  Constant2 : Constant  Value=G1  SampleTime=sampling_time
  Constant3 : Constant  Value=G2  SampleTime=sampling_time
  Constant4 : Constant  Value=I  SampleTime=sampling_time
  Constant5 : Constant  Value=I  SampleTime=sampling_time
  Discrete Derivative : simulink/Discrete/Discrete Derivative  gainval=1.0  ICPrevScaledInput=0.0  OutMin=[]  OutMax=[]  OutDataType=fixdt(1, 16)  OutScaling=2^-10  DoSatur=off
  Drag Plate Aerodynamics : Subsystem
  Gain : Gain
  Gyro : ZeroOrderHold  SampleTime=sampling_time
  Invert 3x3 Matrix1 : aerolibutil/Invert  3x3 Matrix
  Matrix Multiply1 : Product  Multiplication=Matrix(*)
  Matrix Multiply2 : Product  Multiplication=Matrix(*)
  Matrix Multiply3 : Product  Multiplication=Matrix(*)
  Moments due to thrust : MATLAB Function  TreatAsAtomicUnit=on
  Scope : Scope  NumInputPorts=2
  Sum1 : Sum  Inputs=|++
  Vector Concatenate1 : Concatenate  NumInputs=4
  y_model : Outport
  wires:
  Discrete Derivative/1 -> Moments due to thrust/2(omega_dot)
  Constant4/1 -> Invert 3x3 Matrix1/1
  Invert 3x3 Matrix1/1 -> Matrix Multiply3/1, Matrix Multiply2/1, Matrix Multiply1/1
  Moments due to thrust/1(M_t) -> Matrix Multiply3/2, Sum1/1  "thrust_moment_filter"
  [omega_4_f] -> Vector Concatenate1/4
  [omega_2_f] -> Vector Concatenate1/2
  [omega_1_f] -> Vector Concatenate1/1
  [omega_3_f] -> Vector Concatenate1/3
  Sum1/1 -> Matrix Multiply1/2
  Matrix Multiply1/1 -> Gain/1  "pqr_acc_filter"
  Vector Concatenate1/1 -> Moments due to thrust/1(omega), Discrete Derivative/1  "actuators"
  Gyro/1 -> Matrix Multiply2/2, Sum1/2
  Constant3/1 -> Moments due to thrust/4(G2)
  Constant5/1 -> Moments due to thrust/6(I)
  Constant1/1 -> Moments due to thrust/5(sampling_time)
  Constant2/1 -> Moments due to thrust/3(G1)
  Drag Plate Aerodynamics/1(aero_moment) -> Gyro/1  "aero_moment_in"
  Gain/1 -> y_model/1
  Matrix Multiply2/1 -> Scope/1  "pqr_plate"
  Matrix Multiply3/1 -> Scope/2  "pqr_control"

== system B5_simulation_paparazzi/Model Block Complementary Filters/Plant and State Estimation/Complementary Filter ==
  y : Inport
  y_model : Inport  Port=2
  Butterworth Lowpass 2nd Order1 : Subsystem
  Butterworth Lowpass 2nd Order2 : Subsystem
  Scope : Scope  NumInputPorts=3
  Sum : Sum  Inputs=|++
  Sum1 : Sum  Inputs=|+-
  y_est_no_delay : Outport
  wires:
  y/1 -> Butterworth Lowpass 2nd Order1/1(In)  "y"
  Butterworth Lowpass 2nd Order1/1(Out) -> Scope/1, Sum/1  "y_f"
  Butterworth Lowpass 2nd Order2/1(Out) -> Sum1/2, Scope/2  "y_model_f"
  Sum1/1 -> Sum/2  "y_delay_term"
  y_model/1 -> Butterworth Lowpass 2nd Order2/1(In), Sum1/1  "y_model"
  Sum/1 -> Scope/3, y_est_no_delay/1  "y_est_undelayed"

== system B5_simulation_paparazzi/Model Block Complementary Filters/Plant and State Estimation/Complementary Filter1 ==
  y : Inport
  y_model : Inport  Port=2
  Butterworth Lowpass 2nd Order1 : Subsystem
  Butterworth Lowpass 2nd Order2 : Subsystem
  Sum : Sum  Inputs=|++
  Sum1 : Sum  Inputs=|+-
  y_est_no_delay : Outport
  wires:
  y/1 -> Butterworth Lowpass 2nd Order1/1(In)  "y"
  Butterworth Lowpass 2nd Order1/1(Out) -> Sum/1  "y_f"
  Butterworth Lowpass 2nd Order2/1(Out) -> Sum1/2  "y_model_f"
  Sum1/1 -> Sum/2
  y_model/1 -> Butterworth Lowpass 2nd Order2/1(In), Sum1/1  "y_model"
  Sum/1 -> y_est_no_delay/1  "y_est_undelayed"

== system B5_simulation_paparazzi/Model Block Complementary Filters/Plant and State Estimation/Noise Acc ==
  Constant : Constant  Value=NOISE  SampleTime=sampling_time
  Merge : Merge
  Switch Case : SwitchCase
  Switch Case Action Subsystem : Subsystem  TreatAsAtomicUnit=on
  Switch Case Action Subsystem1 : Subsystem  TreatAsAtomicUnit=on
  Out : Outport
  wires:
  Switch Case/2 -> Switch Case Action Subsystem1/Action
  Merge/1 -> Out/1
  Switch Case/1 -> Switch Case Action Subsystem/Action
  Constant/1 -> Switch Case/1
  Switch Case Action Subsystem1/1(Out1) -> Merge/2
  Switch Case Action Subsystem/1(Out1) -> Merge/1

== system B5_simulation_paparazzi/Model Block Complementary Filters/Plant and State Estimation/Noise Gyro ==
  Constant : Constant  Value=NOISE  SampleTime=sampling_time
  Merge : Merge
  Switch Case : SwitchCase
  Switch Case Action Subsystem : Subsystem  TreatAsAtomicUnit=on
  Switch Case Action Subsystem1 : Subsystem  TreatAsAtomicUnit=on
  Out : Outport
  wires:
  Switch Case/2 -> Switch Case Action Subsystem1/Action
  Merge/1 -> Out/1
  Switch Case/1 -> Switch Case Action Subsystem/Action
  Constant/1 -> Switch Case/1
  Switch Case Action Subsystem1/1(Out1) -> Merge/2
  Switch Case Action Subsystem/1(Out1) -> Merge/1

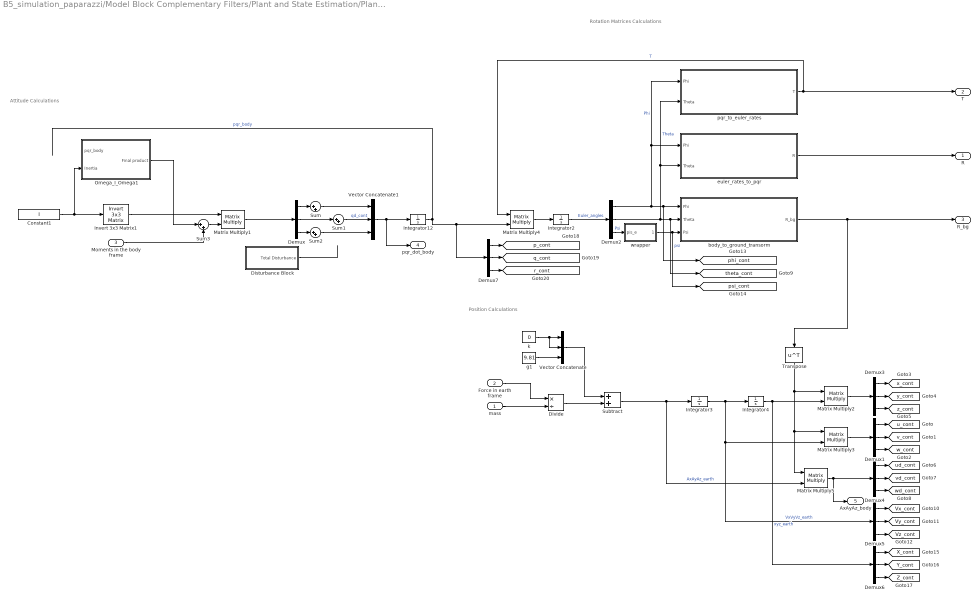
== system B5_simulation_paparazzi/Model Block Complementary Filters/Plant and State Estimation/Plant Dynamics Continuous ==
  note: Attitude Calculations
  note: Rotation Matrices Calculations
  note: Position Calculations
  mass : Inport
  Force in earth frame : Inport  Port=2
  Moments in the body frame : Inport  Port=3
  Constant1 : Constant  Value=I  SampleTime=sampling_time
  Demux{,1..7} (8 alike) : Demux  Outputs=3
  Disturbance Block : Subsystem
  Divide : Product  Inputs=*/
  Integrator{2..4,12} (4 alike) : Integrator
  Invert 3x3 Matrix1 : aerolibutil/Invert  3x3 Matrix
  Matrix Multiply{1..5} (5 alike) : Product  Multiplication=Matrix(*)
  Omega_I_Omega1 : Subsystem
  Subtract : Sum
  Sum{,1..3} (4 alike) : Sum  Inputs=|++
  Transpose : Math  Operator=transpose  SaturateOnIntegerOverflow=on
  Vector Concatenate : Concatenate  NumInputs=3
  Vector Concatenate1 : Concatenate  NumInputs=3
  body_to_ground_transorm : MATLAB Function  Description=|  TreatAsAtomicUnit=on
      | This function computes the rotational matrix to pass from the body frame to the world frame. 
      | Takes as inpout the euler angles.
  euler_rates_to_pqr : MATLAB Function  TreatAsAtomicUnit=on
  g1 : Constant  Value=9.81  VectorParams1D=off
  k : Constant  Value=0  VectorParams1D=off
  pqr_to_euler_rates : MATLAB Function  TreatAsAtomicUnit=on
  wrapper : MATLAB Function  TreatAsAtomicUnit=on
  R : Outport
  T : Outport  Port=2
  R_bg : Outport  Port=3
  pqr_dot_body : Outport  Port=4
  AxAyAz_body : Outport  Port=5
  tag scope: Vx_cont=global, Vy_cont=global, Vz_cont=global, X_cont=global, Y_cont=global, Z_cont=global, p_cont=global, phi_cont=global, psi_cont=global, q_cont=global, r_cont=global, theta_cont=global, u_cont=global, ud_cont=global, v_cont=global, vd_cont=global, w_cont=global, wd_cont=global, x_cont=global, y_cont=global, z_cont=global
  wires:
  Demux/1 -> Sum/1
  Sum2/1 -> Vector Concatenate1/3
  Integrator2/1 -> Demux2/1  "Euler_angles"
  Integrator12/1 -> Demux7/1, Matrix Multiply4/2  "pqr_body"
  Divide/1 -> Subtract/2
  Matrix Multiply5/1 -> AxAyAz_body/1, Demux4/1
  mass/1 -> Divide/2
  Integrator4/1 -> Demux6/1, Matrix Multiply2/2  "xyz_earth"
  Demux2/1 -> pqr_to_euler_rates/1(Phi), euler_rates_to_pqr/1(Phi), [phi_cont], body_to_ground_transorm/1(Phi)  "Phi"
  Vector Concatenate1/1 -> Integrator12/1, pqr_dot_body/1
  Demux/2 -> Sum1/1
  Matrix Multiply3/1 -> Demux1/1
  Demux/3 -> Sum2/1
  Transpose/1 -> Matrix Multiply2/1, Matrix Multiply3/1, Matrix Multiply5/1
  k/1 -> Vector Concatenate/2, Vector Concatenate/1
  Vector Concatenate/1 -> Subtract/1
  pqr_to_euler_rates/1(T) -> T/1, Matrix Multiply4/1  "T"
  Subtract/1 -> Integrator3/1, Matrix Multiply5/2  "AxAyAz_earth"
  Integrator3/1 -> Matrix Multiply3/2, Demux5/1, Integrator4/1  "VxVyVz_earth"
  Matrix Multiply2/1 -> Demux3/1
  Force in earth frame/1 -> Divide/1
  Demux2/3 -> wrapper/1(pis_e)  "Psi"
  Sum/1 -> Vector Concatenate1/1
  Sum1/1 -> Vector Concatenate1/2  "qd_cont"
  body_to_ground_transorm/1(R_bg) -> Transpose/1, R_bg/1
  g1/1 -> Vector Concatenate/3
  Constant1/1 -> Invert 3x3 Matrix1/1, Omega_I_Omega1/2(Inertia)
  Moments in the body frame/1 -> Sum3/2
  euler_rates_to_pqr/1(R) -> R/1
  Invert 3x3 Matrix1/1 -> Matrix Multiply1/1
  Matrix Multiply1/1 -> Demux/1
  Demux1/1 -> [u_cont]
  Demux1/2 -> [v_cont]
  Demux1/3 -> [w_cont]
  Demux3/1 -> [x_cont]
  Demux3/2 -> [y_cont]
  Demux3/3 -> [z_cont]
  Demux4/1 -> [ud_cont]
  Demux4/2 -> [vd_cont]
  Demux4/3 -> [wd_cont]
  Sum3/1 -> Matrix Multiply1/2
  Omega_I_Omega1/1(Final product) -> Sum3/1
  Matrix Multiply4/1 -> Integrator2/1
  Demux2/2 -> [theta_cont], body_to_ground_transorm/2(Theta), pqr_to_euler_rates/2(Theta), euler_rates_to_pqr/2(Theta)  "Theta"
  wrapper/1(psie_w) -> [psi_cont], body_to_ground_transorm/3(Psi)  "psi"
  Demux5/1 -> [Vx_cont]
  Demux5/2 -> [Vy_cont]
  Demux5/3 -> [Vz_cont]
  Demux6/1 -> [X_cont]
  Demux6/2 -> [Y_cont]
  Demux6/3 -> [Z_cont]
  Demux7/1 -> [p_cont]
  Demux7/2 -> [q_cont]
  Demux7/3 -> [r_cont]
  Disturbance Block/1(Total Disturbance) -> ?

== system B5_simulation_paparazzi/Model Block Complementary Filters/Plant and State Estimation/Subsystem1 ==
  Add : Sum
  Constant4 : Constant  Value=K_t  SampleTime=sampling_time
  Forces due to thrust : MATLAB Function  TreatAsAtomicUnit=on
  Gain : Gain  Gain=1/m
  Subtract : Sum
  Terminator : Terminator
  Vector Concatenate : Concatenate  NumInputs=3
  g1 : Constant  Value=9.81  VectorParams1D=off
  k : Constant  Value=0  VectorParams1D=off
  y_model : Outport
  wires:
  Forces due to thrust/1(F_t_e) -> Add/2  "thrust_earth"
  Constant4/1 -> Forces due to thrust/6(K_t)
  [R_bg_discr] -> Forces due to thrust/5(R_bg)
  [omega_1_f] -> Forces due to thrust/1(omega_1)
  [omega_2_f] -> Forces due to thrust/2(omega_2)
  [omega_3_f] -> Forces due to thrust/3(omega_3)
  [omega_4_f] -> Forces due to thrust/4(omega_4)
  Gain/1 -> Subtract/2
  Vector Concatenate/1 -> Subtract/1
  k/1 -> Vector Concatenate/2, Vector Concatenate/1
  g1/1 -> Vector Concatenate/3
  Subtract/1 -> y_model/1  "AxAyAz_earth"
  Add/1 -> Gain/1
  Forces due to thrust/2(F_t_b) -> Terminator/1  "thrust_body"

== system B5_simulation_paparazzi/Model Block Complementary Filters/Simple INDI/8-shape trajectory ==
  Abs : Abs
  Abs1 : Abs
  Clock : Clock
      settings: Decimation=100
  Constant : Constant  Value=f_8
  Constant1 : Constant  Value=scale_8
  Constant2 : Constant  Value=t_8
  Constant3 : Constant  Value=sampling_time
  Constant4 : Constant  Value=0
  Constant5 : Constant  Value=start_8
  Constant6 : Constant  Value=t_8
  Constant7 : Constant  Value=start_8
  Integrator : Integrator
  MATLAB Function : MATLAB Function  TreatAsAtomicUnit=on
  Scope : Scope
  Scope1 : Scope
  Sum : Sum  Inputs=|+-
  Sum3 : Sum  Inputs=|+-
  Sum7 : Sum  Inputs=|+-
  Sum9 : Sum  Inputs=|++
  Switch : Switch  Criteria=u2 > Threshold  Threshold=t_8
  Switch1 : Switch  Criteria=u2 > Threshold  Threshold=start_8
  Zero-Order Hold : ZeroOrderHold  SampleTime=sampling_time
  x_traj : Outport
  y_traj : Outport  Port=2
  psi_traj : Outport  Port=3
  wires:
  Constant2/1 -> Switch/1
  Switch/1 -> Scope/1, MATLAB Function/1(t)  "t"
  Constant/1 -> MATLAB Function/2(f)
  MATLAB Function/2(y) -> y_traj/1, Sum7/2  "y_traj"
  Zero-Order Hold/1 -> Switch/2, Switch/3
  Constant1/1 -> MATLAB Function/3(scale)
  Constant3/1 -> MATLAB Function/4(sampling_time)
  MATLAB Function/1(x) -> x_traj/1, Sum3/2  "x_traj"
  MATLAB Function/3(psi) -> psi_traj/1  "psi_traj"
  Clock/1 -> Sum/1, Switch1/2
  Constant4/1 -> Switch1/3
  Switch1/1 -> Zero-Order Hold/1
  Constant5/1 -> Sum/2
  Sum/1 -> Switch1/1
  Constant6/1 -> MATLAB Function/5(total_time)
  Sum7/1 -> Abs1/1
  Abs/1 -> Sum9/1
  Abs1/1 -> Sum9/2
  [y] -> Sum7/1
  Sum9/1 -> Integrator/1
  Integrator/1 -> Scope1/1  "pos_err"
  [x] -> Sum3/1
  Sum3/1 -> Abs/1
  Constant7/1 -> MATLAB Function/6(start_time)

== system B5_simulation_paparazzi/Model Block Complementary Filters/Simple INDI/Doublet Block ==
  Scope : Scope
  Step : Step  Time=start_time  After=doublet_mag  SampleTime=sampling_time
  theta_cmd : Outport
  wires:
  Step/1 -> theta_cmd/1, Scope/1

== system B5_simulation_paparazzi/Model Block Complementary Filters/Simple INDI/ERROR CONTROLLER ATTITUDE ==
  p_ref : Inport
  q_ref : Inport  Port=2
  r_ref : Inport  Port=3
  phi_ref : Inport  Port=4
  theta_ref : Inport  Port=5
  psi_ref : Inport  Port=6
  Abs : Abs
  Add : Sum  Inputs=++++
  Add1 : Sum  Inputs=++++
  Add2 : Sum  Inputs=+++
  Cumulative Sum : dspmathops/Cumulative Sum  dim=Channels (running sum)  InputProcessing=Columns as channels (frame based)  reset_popup=None  roundingMode=Floor  overflowMode=off  outputDataTypeStr=Inherit: Same as accumulator  outputMin=[]  outputMax=[]  outputLastDataTypeStr=Inherit: Same as accumulator
  Discrete-Time Integrator : DiscreteIntegrator  SampleTime=-1  ICPrevOutput=DiscIntNeverNeededParam  ICPrevScaledInput=DiscIntNeverNeededParam
  Discrete-Time Integrator1 : DiscreteIntegrator  SampleTime=-1  ICPrevOutput=DiscIntNeverNeededParam  ICPrevScaledInput=DiscIntNeverNeededParam
  Discrete-Time Integrator2 : DiscreteIntegrator  SampleTime=-1  ICPrevOutput=DiscIntNeverNeededParam  ICPrevScaledInput=DiscIntNeverNeededParam
  Display : Display
  Display1 : Display
  Gain1 : Gain  Gain=K_ec_d
  Gain10 : Gain  Gain=K_ec_i
  Gain11 : Gain  Gain=K_ec_i
  Gain2 : Gain  Gain=K_ec
  Gain4 : Gain  Gain=K_ec_d
  Gain5 : Gain  Gain=K_ec
  Gain7 : Gain  Gain=K_ec_d
  Gain8 : Gain  Gain=K_ec
  Gain9 : Gain  Gain=K_ec_i
  MATLAB Function1 : MATLAB Function  TreatAsAtomicUnit=on
  Mean : dspstat3/Mean  run=off  InputProcessing=Columns as channels (frame based)  reset_popup=None  directionMode=Each column  dimension=1  roiEnable=off  roiType=Rectangles  roiPortion=Entire ROI  roiOutput=Individual statistics for each ROI  roiFlag=off  roundingMode=Floor  overflowMode=off  outputDataTypeStr=Inherit: Same as accumulator  outputMin=[]  outputMax=[]  outputLastDataTypeStr=Inherit: Same as accumulator
  Sum{1..2,4..5,7..8} (6 alike) : Sum  Inputs=|+-
  pd_ec : Outport
  qd_ec : Outport  Port=2
  rd_ec : Outport  Port=3
  wires:
  p_ref/1 -> Sum1/1
  Add/1 -> pd_ec/1
  [p] -> Sum1/2
  [phi] -> Sum2/2
  phi_ref/1 -> Sum2/1
  Sum1/1 -> Gain1/1  "p_err"
  Sum2/1 -> Discrete-Time Integrator1/1, Gain2/1  "phi_err"
  Gain1/1 -> Add/2
  Gain2/1 -> Add/3
  Sum4/1 -> Gain4/1  "q_err"
  Gain4/1 -> Add1/2
  Gain5/1 -> Add1/3
  theta_ref/1 -> Sum5/1
  [theta] -> Sum5/2
  [q] -> Sum4/2
  q_ref/1 -> Sum4/1
  Add1/1 -> qd_ec/1
  Sum7/1 -> Gain7/1  "r_err"
  Sum8/1 -> MATLAB Function1/1(pis_e)
  Gain7/1 -> Add2/2  "2"
  Gain8/1 -> Add2/3  "3"
  psi_ref/1 -> Sum8/1
  [psi] -> Sum8/2
  [r] -> Sum7/2
  r_ref/1 -> Sum7/1
  Add2/1 -> rd_ec/1
  Sum5/1 -> Abs/1, Discrete-Time Integrator/1, Gain5/1  "theta_err"
  MATLAB Function1/1(psie_w) -> Discrete-Time Integrator2/1, Gain8/1  "psi_err"
  Abs/1 -> Mean/1, Cumulative Sum/1  "theta_err_abs"
  Cumulative Sum/1 -> Display/1
  Mean/1 -> Display1/1
  Discrete-Time Integrator/1 -> Gain9/1
  Gain9/1 -> Add1/4
  Discrete-Time Integrator1/1 -> Gain10/1
  Gain10/1 -> Add/4
  Discrete-Time Integrator2/1 -> Gain11/1
  Gain11/1 -> Add2/1  "4"

== system B5_simulation_paparazzi/Model Block Complementary Filters/Simple INDI/ERROR CONTROLLER VELOCITY ==
  Vx_ref : Inport
  Vy_ref : Inport  Port=2
  Vz_ref : Inport  Port=3
  X_ref : Inport  Port=4
  Y_ref : Inport  Port=5
  Z_ref : Inport  Port=6
  Gain : Gain  Gain=K_ec_u
  Gain1 : Gain  Gain=K_ec_d_u
  Gain2 : Gain  Gain=K_ec_v
  Gain3 : Gain  Gain=K_ec_d_v
  Gain4 : Gain  Gain=K_ec_v
  Gain5 : Gain  Gain=K_ec_d_v
  Sum{,3,5..8} (6 alike) : Sum  Inputs=|+-
  Sum1 : Sum  Inputs=|++
  Sum2 : Sum  Inputs=|++
  Sum4 : Sum  Inputs=|++
  Ax_ec : Outport
  Ay_ec : Outport  Port=2
  Az_ec : Outport  Port=3
  wires:
  [Vz] -> Sum6/2
  Sum1/1 -> Ax_ec/1
  Sum2/1 -> Ay_ec/1
  Vy_ref/1 -> Sum3/1
  Vx_ref/1 -> Sum/1
  [Vy] -> Sum3/2
  Vz_ref/1 -> Sum6/1
  Sum/1 -> Gain1/1  "Vx_error"
  Sum4/1 -> Az_ec/1
  [Vx] -> Sum/2
  [x] -> Sum5/2
  X_ref/1 -> Sum5/1
  Sum5/1 -> Gain/1
  Gain1/1 -> Sum1/1
  Gain/1 -> Sum1/2
  Gain3/1 -> Sum2/1
  Sum3/1 -> Gain3/1  "Vy_error"
  Gain5/1 -> Sum4/1
  Sum6/1 -> Gain5/1  "Vz_error"
  Y_ref/1 -> Sum7/1
  [y] -> Sum7/2
  Sum7/1 -> Gain2/1
  Z_ref/1 -> Sum8/1
  [z] -> Sum8/2
  Sum8/1 -> Gain4/1
  Gain4/1 -> Sum4/2
  Gain2/1 -> Sum2/2
